simulink model "project6"  (R2020b)
settings: Solver=VariableStepAuto  StartTime=0.0  StopTime=10.0  RelTol=1e-3
settings Model: Creator=shrin  LastModifiedBy=shrin

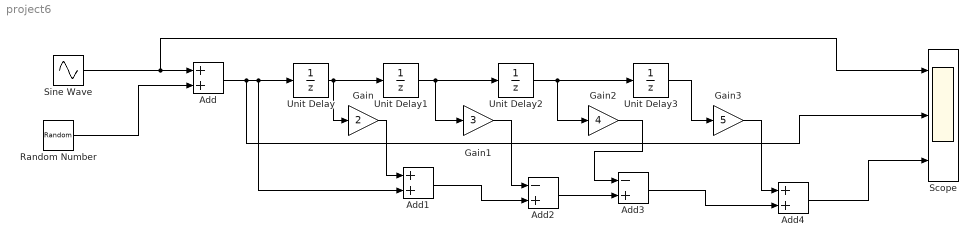
== system project6 ==
  Add : Sum
  Add1 : Sum
  Add2 : Sum  Inputs=-+
  Add3 : Sum  Inputs=-+
  Add4 : Sum
  Gain : Gain  Gain=2
  Gain1 : Gain  Gain=3
  Gain2 : Gain  Gain=4
  Gain3 : Gain  Gain=5
  Random Number : RandomNumber  SampleTime=0.1
  Scope : Scope  NumInputPorts=3
  Sine Wave : Sin  SampleTime=0
  Unit Delay{,1..3} (4 alike) : UnitDelay  SampleTime=-1  HasFrameUpgradeWarning=on
  wires:
  Unit Delay/1 -> Unit Delay1/1, Gain/1
  Unit Delay1/1 -> Gain1/1, Unit Delay2/1
  Unit Delay2/1 -> Gain2/1, Unit Delay3/1
  Unit Delay3/1 -> Gain3/1
  Sine Wave/1 -> Scope/1, Add/1
  Random Number/1 -> Add/2
  Gain/1 -> Add1/1
  Add1/1 -> Add2/2
  Gain1/1 -> Add2/1
  Add2/1 -> Add3/2
  Gain2/1 -> Add3/1
  Gain3/1 -> Add4/1
  Add3/1 -> Add4/2
  Add4/1 -> Scope/3
  Add/1 -> Scope/2, Add1/2, Unit Delay/1
